simulink model "vrmemb1"  (Simulink 6.0)
settings: Solver=VariableStepDiscrete  StartTime=0.0  StopTime=Inf  RelTol=1e-3
PostLoadFcn:
  | vrmemb1_callbacks PostLoad;
libraries: simulink x5, vrlib x1
settings Model: CovMetricSettings=d  Creator=Danek  LastModifiedBy=Houska  ExtModeTrigMode=oneshot  ExtModeArmWhenConnect=off  ExtModeAutoUpdateStatusClock=off
settings DataIOCC: LimitDataPoints=off  SaveOutput=off  SaveTime=off  SignalLoggingName=logsOut
settings OptimizationCC: BlockReduction=off  BooleanDataType=off
settings DebuggingCC: CheckExecutionContextPreStartOutputMsg=on  CheckExecutionContextRuntimeOutputMsg=on  SolverPrmCheckMsg=none
settings HardwareCC: TargetUnknown=on
settings ModelReferenceCC: UpdateModelReferenceTargets=IfOutOfDate
settings GRTTargetCC: LifeSpan=inf
settings SFSimCC: SFSimApplyToAllLibs=on  SFSimBuildMode=Incremental

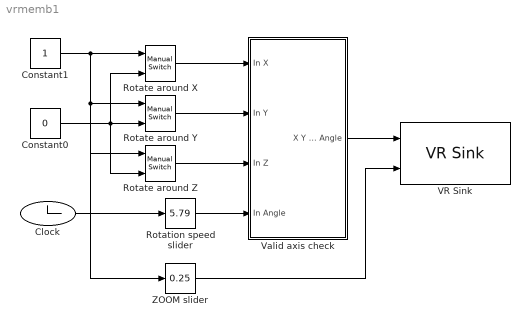
== system vrmemb1 ==
  Clock : Clock
  Constant0 : Constant  Value=0
  Constant1 : Constant
  Rotate around X : simulink/Signal Routing/Manual Switch  sw=0  action=0
  Rotate around Y : simulink/Signal Routing/Manual Switch  sw=0  action=0
  Rotate around Z : simulink/Signal Routing/Manual Switch  sw=1  action=0
  Rotation speed slider : simulink/Math Operations/Slider Gain  low=0  gain=5.79  high=10
  VR Sink : vrlib/VR Sink  SampleTime=0.01  ViewEnable=on  RemoteChange=off  RemoteView=off  FieldsWritten=Membrane.rotation.4.1.double#View1.fieldOfView.1.1.double  WorldFileName=membrane.wrl  AutoView=on
  Valid axis check : Subsystem  Description=This block is used for eliminating the [ 0 0 0 X ] combination of inputs, which would result in undefined rotation.  EnableExecutionContextPropagation=on
  ZOOM slider : simulink/Math Operations/Slider Gain  Description=Use this slider to ZOOM the scene - controls the fieldOfView parameter of View1  low=0.25  gain=0.25  high=0.8
  wires:
  Constant1/1 -> Rotate around X/1, Rotate around Y/1, Rotate around Z/1, ZOOM slider/1
  Constant0/1 -> Rotate around X/2, Rotate around Y/2, Rotate around Z/2
  Rotate around X/1 -> Valid axis check/1(In X)
  Rotate around Y/1 -> Valid axis check/2(In Y)
  Rotate around Z/1 -> Valid axis check/3(In Z)
  Rotation speed slider/1 -> Valid axis check/4(In Angle)
  Clock/1 -> Rotation speed slider/1
  ZOOM slider/1 -> VR Sink/2
  Valid axis check/1(X Y Z Angle) -> VR Sink/1

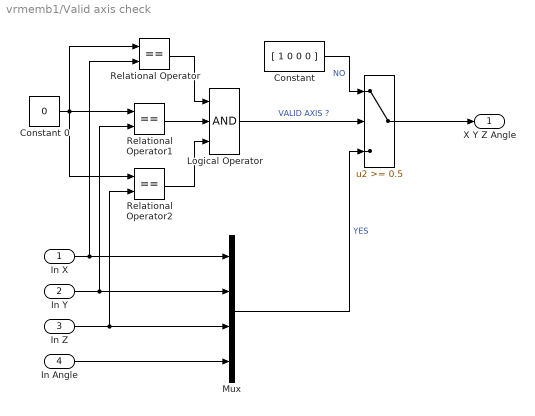
== system vrmemb1/Valid axis check ==
  In X : Inport  LatchInput=off
  In Y : Inport  Port=2  LatchInput=off
  In Z : Inport  Port=3  LatchInput=off
  In Angle : Inport  Port=4  LatchInput=off
  " " : Switch  Threshold=0.5  InputSameDT=on
  Constant : Constant  Value=[ 1 0 0 0 ]
  Constant 0 : Constant  Value=0
  Logical Operator : Logic  Inputs=3
  Mux : Mux
  Relational Operator : RelationalOperator  Operator===  InputSameDT=on
  Relational Operator1 : RelationalOperator  Operator===  InputSameDT=on
  Relational Operator2 : RelationalOperator  Operator===  InputSameDT=on
  X Y Z Angle : Outport
  wires:
  Constant 0/1 -> Relational Operator1/1, Relational Operator2/1, Relational Operator/1
  Relational Operator1/1 -> Logical Operator/2
  Relational Operator2/1 -> Logical Operator/3
  Relational Operator/1 -> Logical Operator/1
  In Z/1 -> Relational Operator2/2, Mux/3
  In Y/1 -> Relational Operator1/2, Mux/2
  In X/1 -> Relational Operator/2, Mux/1
  Mux/1 -> " "/3  "YES"
  Logical Operator/1 -> " "/2  "VALID AXIS ?"
  In Angle/1 -> Mux/4
  " "/1 -> X Y Z Angle/1
  Constant/1 -> " "/1  "NO"
